simulink model "duffing_plant"  (R2018a)
settings: Solver=FixedStepAuto  StartTime=0.0  StopTime=tsim  FixedStep=hsim  RelTol=1e-3
values from neighbouring files (symbols this model uses):
  alpha = -1    [init.m]
  beta = 1    [init.m]
  delta = 0.3    [init.m]
  hsim = 0.001    [init.m]
  noise_on = 0    [init.m]
  omega_d = 1.2    [init.m]
  var = 0.00001    (= 1e-05)    [init.m]
  x1_init = 1    [init.m]
  x2_init = 0    [init.m]
undefined symbols (not defined in the file or in its folder): gamma
settings Model: Creator=giulio  LastModifiedBy=giulio
settings ModelReferenceCC: ModelReferenceNumInstancesAllowed=Single

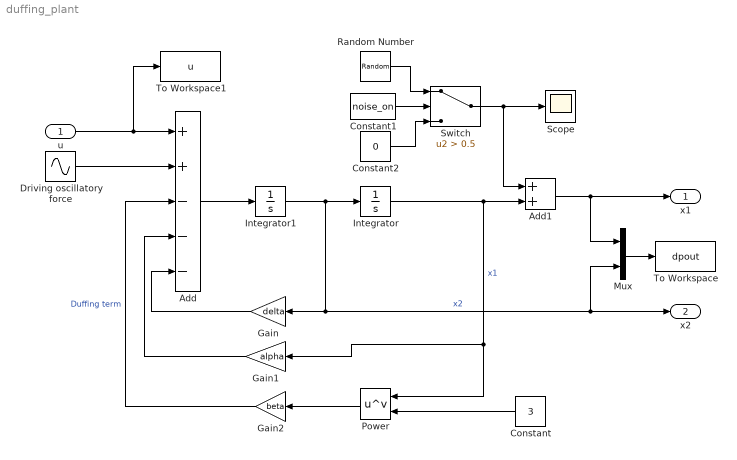
== system duffing_plant ==
  u : Inport
  Add : Sum  Inputs=++---
  Add1 : Sum  Inputs=2
  Constant : Constant  Value=3
  Constant1 : Constant  Value=noise_on
  Constant2 : Constant  Value=0
  Driving oscillatory force : Sin  Amplitude=gamma  Frequency=omega_d  Phase=pi/2  SampleTime=0
  Gain : Gain  Gain=delta
  Gain1 : Gain  Gain=alpha
  Gain2 : Gain  Gain=beta
  Integrator : Integrator  InitialCondition=x1_init
  Integrator1 : Integrator  InitialCondition=x2_init
  Mux : Mux  Inputs=2
  Power : Math  Operator=pow  SaturateOnIntegerOverflow=on
  Random Number : RandomNumber  Variance=var  SampleTime=hsim
  Scope : Scope
  Switch : Switch  Criteria=u2 > Threshold  Threshold=0.5
  To Workspace : ToWorkspace  VariableName=dpout  SampleTime=-1
  To Workspace1 : ToWorkspace  VariableName=u  SampleTime=-1
  x1 : Outport
  x2 : Outport  Port=2
  wires:
  Integrator/1 -> Power/1, Gain1/1, Add1/2  "x1"
  Integrator1/1 -> Mux/2, x2/1, Gain/1, Integrator/1  "x2"
  Add/1 -> Integrator1/1
  Gain/1 -> Add/5
  Driving oscillatory force/1 -> Add/2
  Gain1/1 -> Add/4
  Gain2/1 -> Add/3  "Duffing term"
  Power/1 -> Gain2/1
  Constant/1 -> Power/2
  u/1 -> To Workspace1/1, Add/1
  Constant1/1 -> Switch/2
  Random Number/1 -> Switch/1
  Constant2/1 -> Switch/3
  Add1/1 -> Mux/1, x1/1
  Switch/1 -> Add1/1, Scope/1
  Mux/1 -> To Workspace/1
